simulink model "Project1DigiCont"  (R2017b)
settings: Solver=VariableStepAuto  StartTime=0.0  StopTime=inf  RelTol=1e-3
libraries: realtime_pacer_lib x1
settings Model: Creator=segadiallo  LastModifiedBy=segadiallo

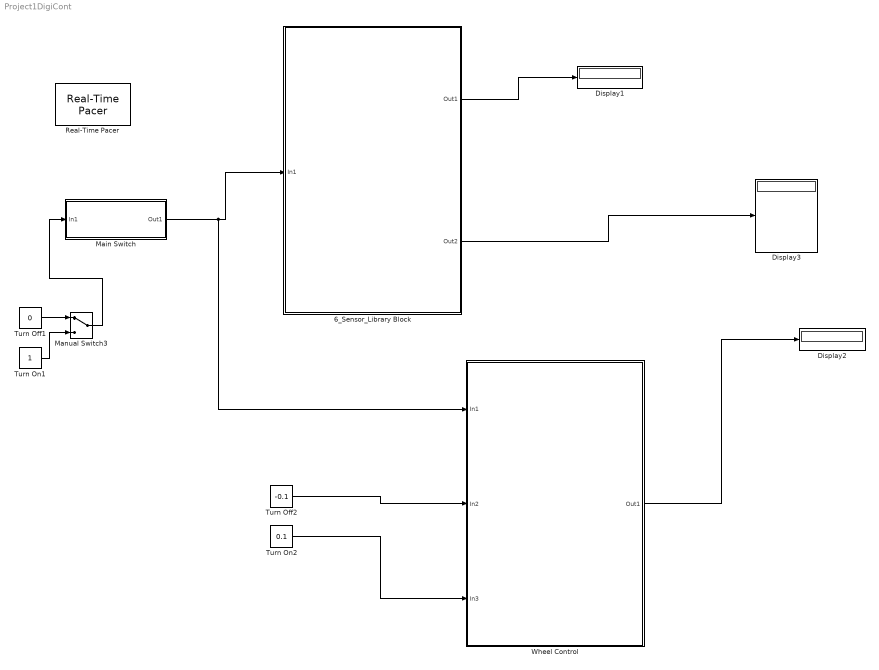
== system Project1DigiCont ==
  6_Sensor_Library Block : Subsystem
      mask help: Six sensor test
      mask Display:
      | disp('6_Sensors_Test')
      | port_label('output',1,'Status')
      | port_label('output',2,'display')
      | port_label('input',1,'InputV')
  Display1 : Display
  Display2 : Display
  Display3 : Display
  Main Switch : Subsystem
      mask Display:
      | disp('Main Switch')
      | port_label('output',1,'inputV')
      | port_label('input',1,'Go')
  Manual Switch3 : ManualSwitch
  Real-Time Pacer : realtime_pacer_lib/Real-Time Pacer  simTimePerRealTime=1
  Turn Off1 : Constant  Value=0
  Turn Off2 : Constant  Value=-0.1
  Turn On1 : Constant
  Turn On2 : Constant  Value=0.1
  Wheel Control : Subsystem
      mask Display:
      | disp('Wheel Controle');
      | port_label('output',1,'Status');
      | port_label('input',2,'rightW');
      | port_label('input',1,'InputV');
      | port_label('input',3,'leftW');
  wires:
  Wheel Control/1(Out1) -> Display2/1
  6_Sensor_Library Block/1(Out1) -> Display1/1
  6_Sensor_Library Block/2(Out2) -> Display3/1
  Turn Off1/1 -> Manual Switch3/1
  Turn On1/1 -> Manual Switch3/2
  Manual Switch3/1 -> Main Switch/1(In1)
  Main Switch/1(Out1) -> Wheel Control/1(In1), 6_Sensor_Library Block/1(In1)
  Turn On2/1 -> Wheel Control/3(In3)
  Turn Off2/1 -> Wheel Control/2(In2)

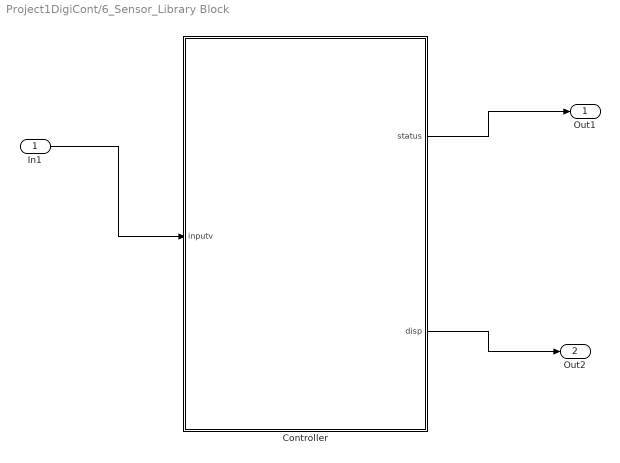
== system Project1DigiCont/6_Sensor_Library Block ==
  In1 : Inport
  Controller : Stateflow chart  TreatAsAtomicUnit=on
  Out1 : Outport
  Out2 : Outport  Port=2
  wires:
  In1/1 -> Controller/1(inputv)
  Controller/1(status) -> Out1/1
  Controller/2(disp) -> Out2/1

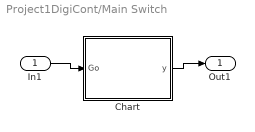
== system Project1DigiCont/Main Switch ==
  In1 : Inport
  Chart : Stateflow chart  TreatAsAtomicUnit=on
  Out1 : Outport
  wires:
  Chart/1(y) -> Out1/1
  In1/1 -> Chart/1(Go)

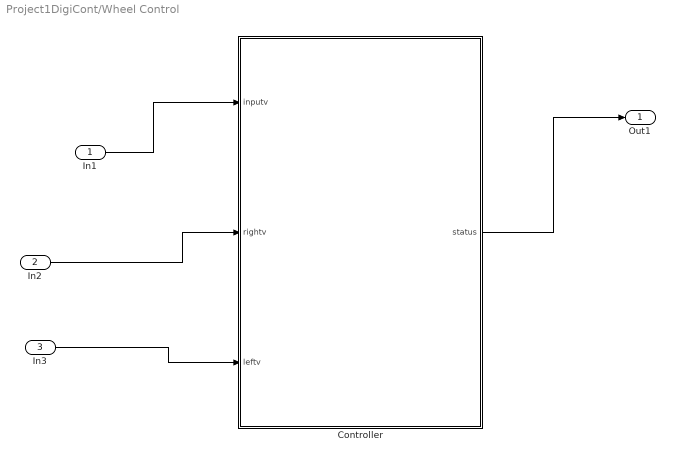
== system Project1DigiCont/Wheel Control ==
  In1 : Inport
  In2 : Inport  Port=2
  In3 : Inport  Port=3
  Controller : Stateflow chart  TreatAsAtomicUnit=on
  Out1 : Outport
  wires:
  Controller/1(status) -> Out1/1
  In3/1 -> Controller/3(leftv)
  In2/1 -> Controller/2(rightv)
  In1/1 -> Controller/1(inputv)

== stateflow chart Project1DigiCont/Wheel Control/Controller ==
  state NoCommand
    entry:
    status=0
  state Start
    during:
    entry:
    coder.extrinsic('evalin');
    obj = evalin('base','objWs');
    SetWheelVelRoomba(obj, rightv, leftv)
    status = 1;
  state Reset
  (default) -> NoCommand
  NoCommand -> Start : [inputv==2 ]
  Start -> Start [order 2] : after(0.1,sec)
  Reset -> Start : [inputv==2]
  Start -> Reset [order 1] : [inputv~=1]
  data: inputv input size=1; status output; so local; rightv input; leftv input; obj local

== stateflow chart Project1DigiCont/Main Switch/Chart ==
  state START
    entry:
    y=0
  state CONNECT
    entry: tcpInit;
  state DISCONNECT
    entry: y=0
    coder.extrinsic('evalin')
    obj=evalin('base','objWs')
    fclose(obj)
  state Toggle
    entry: y = y + 1
    if y==3
    y=1
    end
  state SerialControl1
    entry: y==1
  (default) -> START
  START -> CONNECT : [Go==1]
  DISCONNECT -> CONNECT : [Go==1]
  CONNECT -> DISCONNECT [order 1] : [Go==0]
  SerialControl1 -> DISCONNECT [order 2] : [Go ==0]
  CONNECT -> SerialControl1 [order 2]
  Toggle -> SerialControl1 : after(1,sec)
  SerialControl1 -> Toggle [order 1] : [Go==1]
  data: Go input; obj local; y output
  function tcpInit:
    | function tcpInit
    | coder.extrinsic('tcpip');
    | coder.extrinsic('assignin');
    | persistent obj
    | 
    | serPort = tcpip('10.0.0.1',9001);
    | set(serPort,'Terminator','LF')
    | set(serPort,'InputBufferSize',1000)
    | set(serPort, 'Timeout', .5)
    | set(serPort, 'ByteOrder','bigEndian');
    | 
    | fopen(serPort);
    | 
    | Start=[128];
    | fwrite(serPort,Start);
    | pause(.1)
    | Mode= 132;
    | fwrite(serPort,Mode);
    | pause(.1)
    | 
    | % %Print 'go' on display
    | fwrite(serPort, [164, 71, 79, 32, 32]);
    | % make a sound
    | fwrite(serPort, [140 1 3 60 20 72 20 84 40 ]); %RoombaInit Song
    | fwrite(serPort, [140 2 1 60 20]); % BeepRoomba song
    | fwrite(serPort, [140 3 3 84 20 72 30 60 40]); % PowerOffRoomba song
    | fwrite(serPort, [141 1]); % play RoombaInit song
    | 
    | obj=serPort;
    | 
    | assignin('base','objWs',obj);
    | end

== stateflow chart Project1DigiCont/6_Sensor_Library Block/Controller ==
  state init
    entry:
    coder.extrinsic('evalin');
    obj = evalin('base','objWs');
    disp=[nan;0;0;0;0;0];
    status = 0
  state NoCommand
    entry:
    disp=[0;0;0;0;0;0];
    status=0
  state Start
    entry:
    coder.extrinsic('evalin');
    obj = evalin('base','objWs');
    coder.extrinsic('RangeStateRoomba')
    disp=RangeStateRoomba(obj);
    status = 1;
  (default) -> NoCommand
  NoCommand -> init : after(0.5,sec)[inputv==1]
  init -> Start : [inputv==1]
  Start -> init [order 2] : [inputv~=1]
  Start -> Start [order 1] : after(0.1,sec)
  data: inputv input size=1; status output; so local; disp output double size=6; obj local
